simulink model "q_aero_attitude"  (Simulink 10.0)
settings: Solver=ode1  StartTime=0.0  StopTime=30  FixedStep=0.002  RelTol=1e-3  EnableMultiTasking=on
undefined symbols (not defined in the file or in its folder): HIL, qc_get_step_size
libraries: quarc_library x4, simulink_extras x2
settings Model: Creator=MLevis  LastModifiedBy=johannes  SimulationMode=external  ExtModeTrigDuration=20000
settings SolverCC: PositivePriorityOrder=on
settings DataIOCC: LimitDataPoints=on  SignalLoggingSaveFormat=ModelDataLogs
settings OptimizationCC: ExpressionDepthLimit=2147483647
settings DebuggingCC: SolverPrmCheckMsg=warning  FcnCallInpInsideContextMsg=warning  StateNameClashWarn=warning
settings RTWCC: Description=QUARC Win64 Target  SystemTargetFile=quarc_win64.tlc  TemplateMakefile=quarc_default_tmf
settings STFCustomTargetCC: TargetPreCompLibLocation=C:\PROGRA~3\QUARC\lib\2014a\win64\release  ConcurrentExecutionCompliant=on  GeneratePreprocessorConditionals=Disable all  CombineOutputUpdateFcns=on  CPPClassGenCompliant=on  GRTInterface=off  SystemTargetFile=quarc_win64.tlc
settings GRTTargetCC: TargetPreCompLibLocation=C:\PROGRA~3\QUARC\lib\2014a\win64\release  ParMdlRefBuildCompliant=off  CompOptLevelCompliant=off  GeneratePreprocessorConditionals=Disable all  CombineOutputUpdateFcns=on  MatFileLogging=off  GRTInterface=off  UseToolchainInfoCompliant=off  ExtMode=on  ExtModeMexFile=quarc_comm
settings ConfigComp: CovExternalEMLEnable=off  CovSFcnEnable=off

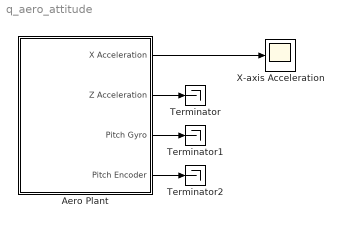
== system q_aero_attitude ==
  Aero Plant : Subsystem
  Terminator : Terminator
  Terminator1 : Terminator
  Terminator2 : Terminator
  X-axis Acceleration : Scope
  wires:
  Aero Plant/1(X Acceleration) -> X-axis Acceleration/1
  Aero Plant/2(Z Acceleration) -> Terminator/1
  Aero Plant/3(Pitch Gyro) -> Terminator1/1
  Aero Plant/4(Pitch Encoder) -> Terminator2/1

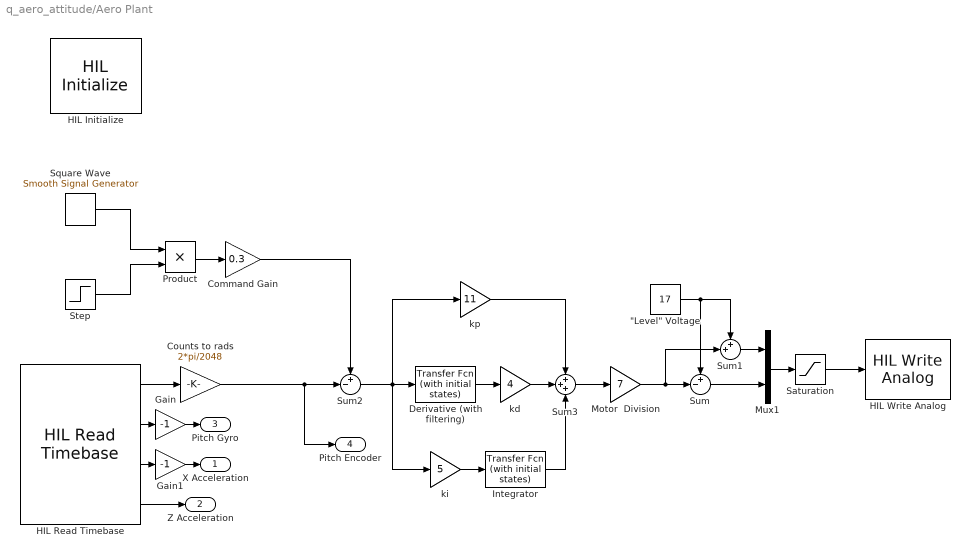
== system q_aero_attitude/Aero Plant ==
  "\"Level\" Voltage" : Constant  Value=17
  Command Gain : Gain  Gain=0.3
  Counts to rads : Gain  Gain=2*pi/2048
  Derivative (with filtering) : simulink_extras/Additional Linear/Transfer Fcn (with initial states)  N=[20 0]  D=[1 20]  X0=0
  Gain : Gain  Gain=-1
  Gain1 : Gain  Gain=-1
  HIL Initialize : quarc_library/Data Acquisition/Generic/Configuration/HIL Initialize  Priority=-99  object_name=HIL-1  board_type=quanser_aero_usb  board_number=0  board_options=""  exclusive=off  active=off  hardware_clocks=[0]  clock_modes=[]  initial_clock_frequencies=[]  set_clock_params_at_start=off  set_clock_params_at_switch_in=off  set_clock_frequencies_at_start=off  set_clock_frequencies_at_switch_in=off  analog_input_channels=[0:1]  analog_input_maximums=3  analog_input_minimums=-3  set_analog_input_params_at_start=off  set_analog_input_params_at_switch_in=off  analog_output_channels=[0:1]  analog_output_maximums=24  analog_output_minimums=-24  initial_analog_outputs=[0]  final_analog_outputs=[0]  watchdog_analog_outputs=[0]  set_analog_output_params_at_start=off  set_analog_output_params_at_switch_in=off  set_analog_outputs_at_start=on  set_analog_outputs_at_switch_in=off  set_analog_outputs_at_terminate=on  set_analog_outputs_at_switch_out=off  set_analog_outputs_on_watchdog=off  digital_input_channels=[]  digital_output_channels=[0:1]  digital_output_configuration=[]  initial_digital_outputs=[1]  final_digital_outputs=[0]  watchdog_digital_outputs=[0]  set_digital_output_params_at_start=off  set_digital_output_params_at_switch_in=off  set_digital_outputs_at_start=on  set_digital_outputs_at_switch_in=off  set_digital_outputs_at_terminate=on  set_digital_outputs_at_switch_out=off  set_digital_outputs_on_watchdog=off  encoder_channels=[0:3]  quadrature=[4]  encoder_filter_frequency=[]  initial_encoder_counts=[0]  set_encoder_params_at_start=off  set_encoder_params_at_switch_in=off  set_encoder_counts_at_start=on  set_encoder_counts_at_switch_in=off  pwm_channels=[]  pwm_modes=[]  pwm_frequency=[]  pwm_configuration=[]  pwm_alignment=[]  pwm_polarity=[]  pwm_leading_deadband=[]  pwm_trailing_deadband=[]  initial_pwm_outputs=[]  final_pwm_outputs=[]  watchdog_pwm_outputs=[]  set_pwm_params_at_start=off  set_pwm_params_at_switch_in=off  set_pwm_outputs_at_start=off  set_pwm_outputs_at_switch_in=off  set_pwm_outputs_at_terminate=off  set_pwm_outputs_at_switch_out=off  set_pwm_outputs_on_watchdog=off  other_output_channels=[11000:11002]  initial_other_outputs=[0 1 0]  final_other_outputs=[1 0 0]  watchdog_other_outputs=[0 0 1]  set_other_outputs_at_start=on  set_other_outputs_at_switch_in=off  set_other_outputs_at_terminate=on  set_other_outputs_at_switch_out=off  set_other_outputs_on_watchdog=off
  HIL Read Timebase : quarc_library/Data Acquisition/Generic/Timebases/HIL Read Timebase  object_name=HIL-1  clock=0  analog_channels=[]  encoder_channels=[2]  digital_channels=[]  other_channels=[3001 4000 4002]  samples_in_buffer=max(ceil(1/qc_get_step_size), 1)  active=on  vector_output=off  data_type_mode=Inherit via back propagation  encoder_data_type=double  digital_data_type=boolean
  HIL Write Analog : quarc_library/Data Acquisition/Generic/Immediate I//O/HIL Write Analog  object_name=HIL-1  channels=[0:1]  sample_time=-1  active=off  vector_input=on
  Integrator : simulink_extras/Additional Linear/Transfer Fcn (with initial states)  N=[1]  D=[1 0]  X0=0
  Motor  Division : Gain  Gain=7
  Mux1 : Mux  Inputs=2
  Product : Product
  Saturation : Saturate  UpperLimit=24  LowerLimit=10
  Square Wave : quarc_library/Sources/Signals/Smooth Signal Generator  signal_type=Square  source=Internal (dialog parameters)  amplitude=1  frequency=0.1  initial_phase=pi  sample_time=qc_get_step_size  output_cos=off
  Step : Step  Time=5  SampleTime=0
  Sum : Sum  Inputs=+-|
  Sum1 : Sum  Inputs=++|
  Sum2 : Sum  Inputs=+-|
  Sum3 : Sum  Inputs=+++
  kd : Gain  Gain=4
  ki : Gain  Gain=5
  kp : Gain  Gain=11
  X Acceleration : Outport
  Z Acceleration : Outport  Port=2
  Pitch Gyro : Outport  Port=3
  Pitch Encoder : Outport  Port=4
  wires:
  HIL Read Timebase/1 -> Counts to rads/1
  "\"Level\" Voltage"/1 -> Sum1/1, Sum/1
  Sum/1 -> Mux1/2
  Sum1/1 -> Mux1/1
  Motor  Division/1 -> Sum1/2, Sum/2
  Command Gain/1 -> Sum2/1
  Counts to rads/1 -> Sum2/2, Pitch Encoder/1
  Sum2/1 -> ki/1, Derivative (with filtering)/1, kp/1
  kp/1 -> Sum3/1
  Derivative (with filtering)/1 -> kd/1
  kd/1 -> Sum3/2
  ki/1 -> Integrator/1
  Integrator/1 -> Sum3/3
  Sum3/1 -> Motor  Division/1
  Mux1/1 -> Saturation/1
  Saturation/1 -> HIL Write Analog/1
  Product/1 -> Command Gain/1
  Square Wave/1 -> Product/1
  Step/1 -> Product/2
  HIL Read Timebase/2 -> Gain/1
  HIL Read Timebase/3 -> Gain1/1
  HIL Read Timebase/4 -> Z Acceleration/1
  Gain/1 -> Pitch Gyro/1
  Gain1/1 -> X Acceleration/1
